simulink model "CT_T1_val"  (Simulink 7.0)
settings: Solver=FixedStepDiscrete  StartTime=0.0  StopTime=60  FixedStep=0.1  RelTol=1e-3
undefined symbols (not defined in the file or in its folder): A, B
settings Model: Creator=Equipo-Servo  LastModifiedBy=Equipo-Servo  ExtModeTrigDuration=100000
settings OptimizationCC: InitFltsAndDblsToZero=off
settings DebuggingCC: AlgebraicLoopMsg=none  FcnCallInpInsideContextMsg=Enable All  StrictBusMsg=ErrorLevel1
settings HardwareCC: ProdIntDivRoundTo=Zero  ProdEndianess=LittleEndian  ProdHWDeviceType=Generic->32-bit x86 compatible
settings RTWCC: SystemTargetFile=rtwin.tlc  TemplateMakefile=rtwin.tmf  Description=Real-Time Windows Target  ProcessScript=rtwin_make_rtw_hook  RTWCompilerOptimization=On
settings CodeAppCC: MaxIdLength=95  CustomSymbolStrType=$N$R$M_T
settings RTWinTargetCC: TargetLibSuffix=_rtwin.lib  TargetPreCompLibLocation=C:\Program Files\MATLAB\R2013a\toolbox\rtw\targets\rtwin\lib\win32  GenFloatMathFcnCalls=ANSI_C  MatFileLogging=on  RTWinDir=C:/PROGRA~1/MATLAB/R2013a/toolbox/rtw/targets/rtwin  TargetArch=win32

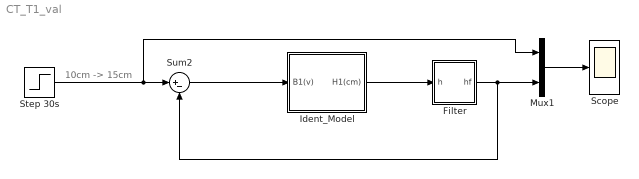
== system CT_T1_val ==
  note: 10cm -> 15cm
  Filter : Subsystem  mask{O=1, Fc=0.5}
      mask prompts: O "Orden"; Fc "Frecuencia de corte"
      mask init:
      | [B,A] = butter(O,Fc/(10/2));
  Ident_Model : Subsystem
  Mux1 : Mux  Inputs=2
  Scope : Scope
      settings: TimeRange=100  YMin=0  YMax=30
  Step 30s : Step  Time=30  Before=10  After=15  SampleTime=0
  Sum2 : Sum  Inputs=|+-
  wires:
  Step 30s/1 -> Mux1/1, Sum2/1
  Mux1/1 -> Scope/1
  Ident_Model/1(H1(cm)) -> Filter/1(h)
  Filter/1(hf) -> Mux1/2, Sum2/2
  Sum2/1 -> Ident_Model/1(B1(v))

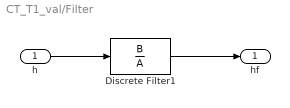
== system CT_T1_val/Filter ==
  h : Inport
  Discrete Filter1 : DiscreteFilter  Numerator=B  Denominator=A  SampleTime=0.1
  hf : Outport
  wires:
  Discrete Filter1/1 -> hf/1
  h/1 -> Discrete Filter1/1

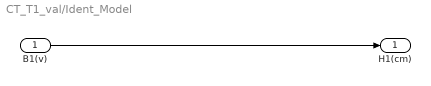
== system CT_T1_val/Ident_Model ==
  B1(v) : Inport
  H1(cm) : Outport
  wires:
  B1(v)/1 -> H1(cm)/1
